simulink model "Takeoff_Sim"  (R2024a)
settings: Solver=ode4  StartTime=0.0  StopTime=15  FixedStep=0.01  RelTol=1e-3
values from neighbouring files (symbols this model uses):
  alpha_L0 = deg2rad(-2)    [Takeoff_Script.m]
  carrier_vel = 25 * 0.5144444444    (= 12.86111111)    [Takeoff_Script.m]
  CD_0 = 0.025    [Takeoff_Script.m]
  CD_LG = 0.01    [Takeoff_Script.m]
  CL_alpha = 2 * pi * AR / (2 + sqrt(AR^2 + 4))    [Takeoff_Script.m]
  g_accel = 9.807    [Takeoff_Script.m]
  k_drag = 1.0 / (eswald * pi * AR)    [Takeoff_Script.m]
  mass = 14000    [Takeoff_Script.m]
  mu_friction_nobrake = 0.04    [Takeoff_Script.m]
  thrust = 10000 * g_accel    (= 98070)    [Takeoff_Script.m]
  wingarea = x(1)    [Takeoff_Script.m]
libraries: simulink_extras x5, aerolibasang x2, aerolibatmos2 x1
settings Model: Creator=mfarr  LastModifiedBy=mfarr
settings OptimizationCC: BlockReduction=off  DefaultParameterBehavior=Inlined  BufferReuse=off

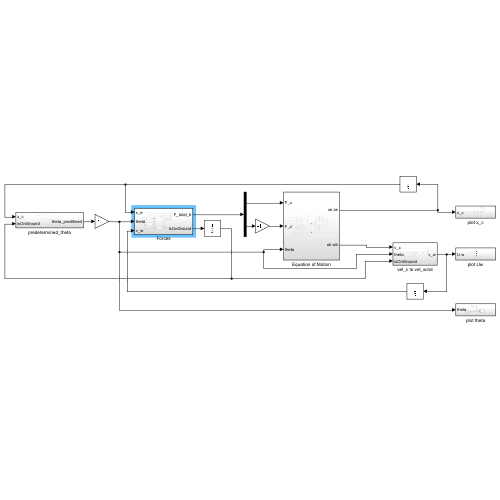
[thumbnail: Simulink's stored preview of the top-level diagram]
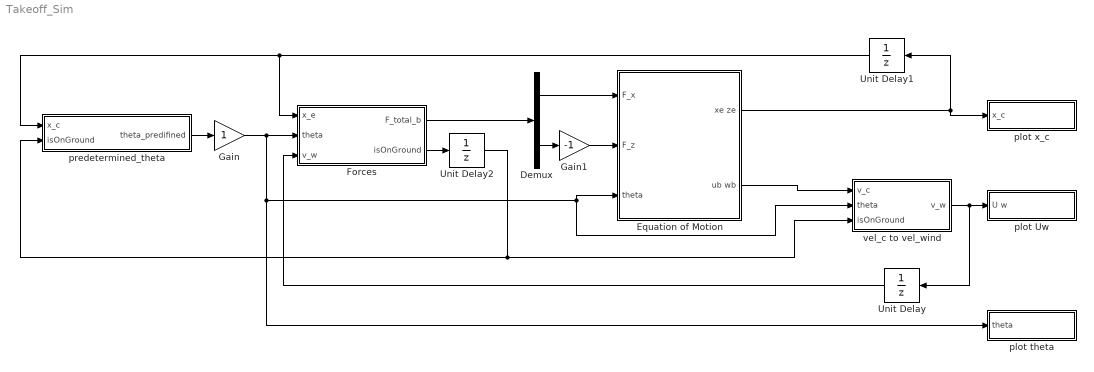
== system Takeoff_Sim ==
  Demux : Demux  Outputs=2
  Equation of Motion : Subsystem
  Forces : Subsystem
  Gain : Gain
  Gain1 : Gain  Gain=-1
  Unit Delay : UnitDelay  SampleTime=-1  HasFrameUpgradeWarning=on
  Unit Delay1 : UnitDelay  SampleTime=-1  HasFrameUpgradeWarning=on
  Unit Delay2 : UnitDelay  SampleTime=-1  HasFrameUpgradeWarning=on
  plot Uw : Subsystem
  plot theta : Subsystem
  plot x_c : Subsystem
  predetermined_theta : Subsystem
  vel_c to vel_wind : Subsystem
  wires:
  vel_c to vel_wind/1(v_w) -> Unit Delay/1, plot Uw/1(U w)
  Equation of Motion/2(ub wb) -> vel_c to vel_wind/1(v_c)
  Demux/1 -> Equation of Motion/1(F_x)
  Forces/1(F_total_b) -> Demux/1
  predetermined_theta/1(theta_predifined) -> Gain/1
  Unit Delay/1 -> Forces/3(v_w)
  Unit Delay1/1 -> predetermined_theta/1(x_c), Forces/1(x_e)
  Forces/2(isOnGround) -> Unit Delay2/1
  Unit Delay2/1 -> predetermined_theta/2(isOnGround), vel_c to vel_wind/3(isOnGround)
  Gain/1 -> Forces/2(theta), vel_c to vel_wind/2(theta), Equation of Motion/3(theta), plot theta/1(theta)
  Demux/2 -> Gain1/1
  Gain1/1 -> Equation of Motion/2(F_z)
  Equation of Motion/1(xe ze) -> plot x_c/1(x_c), Unit Delay1/1

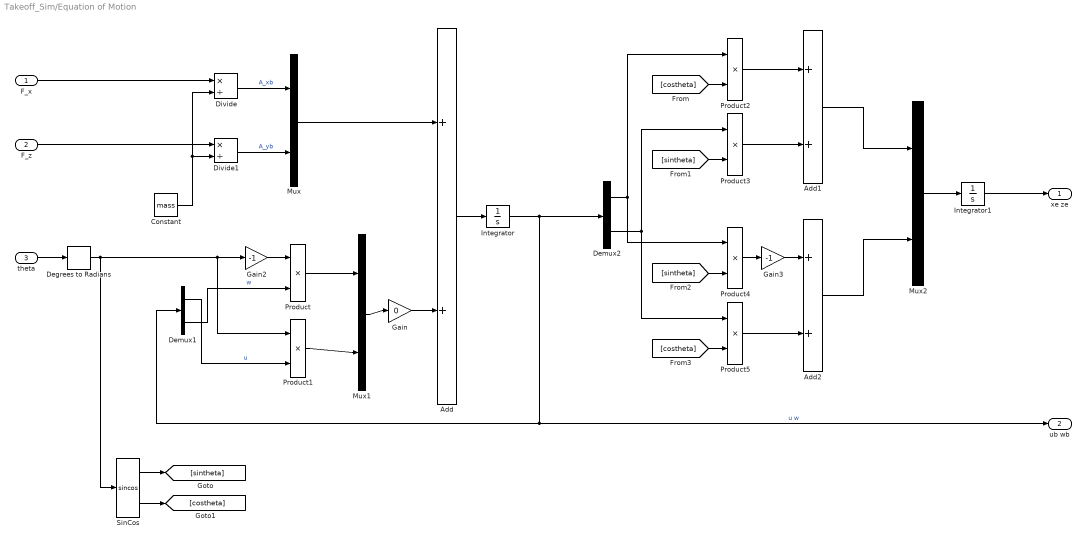
== system Takeoff_Sim/Equation of Motion ==
  F_x : Inport
  F_z : Inport  Port=2
  theta : Inport  Port=3
  Add : Sum
  Add1 : Sum
  Add2 : Sum
  Constant : Constant  Value=mass
  Degrees to Radians : simulink_extras/Transformations/Degrees to Radians
  Demux1 : Demux  Outputs=2
  Demux2 : Demux  Outputs=2
  Divide : Product  Inputs=*/  RndMeth=Zero  SaturateOnIntegerOverflow=on
  Divide1 : Product  Inputs=*/  RndMeth=Zero  SaturateOnIntegerOverflow=on
  Gain : Gain  Gain=0
  Gain2 : Gain  Gain=-1
  Gain3 : Gain  Gain=-1
  Integrator : Integrator
  Integrator1 : Integrator
  Mux : Mux  Inputs=2
  Mux1 : Mux  Inputs=2
  Mux2 : Mux  Inputs=2
  Product{,1..5} (6 alike) : Product
  SinCos : Trigonometry  Operator=sincos
  xe ze : Outport
  ub wb : Outport  Port=2
  wires:
  Demux1/2 -> Product/2  "w"
  Add1/1 -> Mux2/1
  SinCos/2 -> [costheta]
  Degrees to Radians/1 -> Product1/1, Gain2/1, SinCos/1
  Gain2/1 -> Product/1
  Divide1/1 -> Mux/2  "A_yb"
  Add/1 -> Integrator/1
  Mux/1 -> Add/1
  Demux1/1 -> Product1/2  "u"
  theta/1 -> Degrees to Radians/1
  Integrator/1 -> Demux2/1, ub wb/1, Demux1/1  "u w"
  Product5/1 -> Add2/2
  [costheta] -> Product5/2
  [costheta] -> Product2/2
  Product4/1 -> Gain3/1
  Mux1/1 -> Gain/1
  Constant/1 -> Divide1/2, Divide/2
  Demux2/2 -> Product3/1, Product5/1
  Divide/1 -> Mux/1  "A_xb"
  Mux2/1 -> Integrator1/1
  F_z/1 -> Divide1/1
  SinCos/1 -> [sintheta]
  [sintheta] -> Product3/2
  Demux2/1 -> Product4/1, Product2/1
  Gain3/1 -> Add2/1
  [sintheta] -> Product4/2
  Product3/1 -> Add1/2
  Integrator1/1 -> xe ze/1
  Product1/1 -> Mux1/2
  Product/1 -> Mux1/1
  Product2/1 -> Add1/1
  Add2/1 -> Mux2/2
  F_x/1 -> Divide/1
  Gain/1 -> Add/2

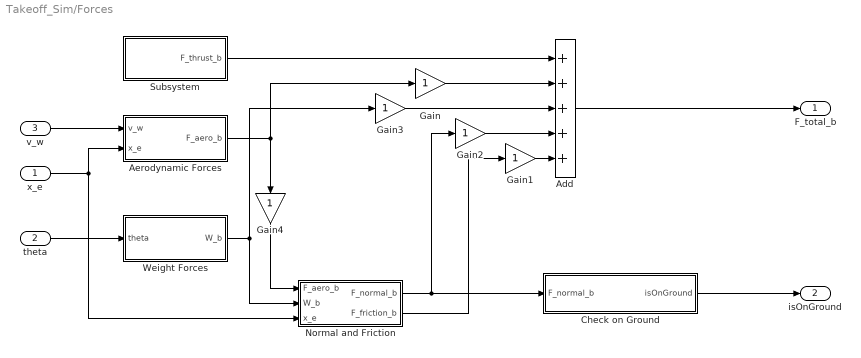
== system Takeoff_Sim/Forces ==
  x_e : Inport
  theta : Inport  Port=2
  v_w : Inport  Port=3
  Add : Sum  Inputs=+++++
  Aerodynamic Forces : Subsystem
  Check on Ground : Subsystem
  Gain{,1..4} (5 alike) : Gain
  Normal and Friction : Subsystem
  Subsystem : Subsystem
  Weight Forces : Subsystem
  F_total_b : Outport
  isOnGround : Outport  Port=2
  wires:
  Aerodynamic Forces/1(F_aero_b) -> Gain/1, Gain4/1
  Weight Forces/1(W_b) -> Gain3/1, Normal and Friction/2(W_b)
  theta/1 -> Weight Forces/1(theta)
  v_w/1 -> Aerodynamic Forces/1(v_w)
  x_e/1 -> Normal and Friction/3(x_e), Aerodynamic Forces/2(x_e)
  Add/1 -> F_total_b/1
  Subsystem/1(F_thrust_b) -> Add/1
  Normal and Friction/1(F_normal_b) -> Check on Ground/1(F_normal_b), Gain2/1
  Normal and Friction/2(F_friction_b) -> Gain1/1
  Gain/1 -> Add/2
  Gain1/1 -> Add/5
  Gain2/1 -> Add/4
  Gain3/1 -> Add/3
  Check on Ground/1(isOnGround) -> isOnGround/1
  Gain4/1 -> Normal and Friction/1(F_aero_b)

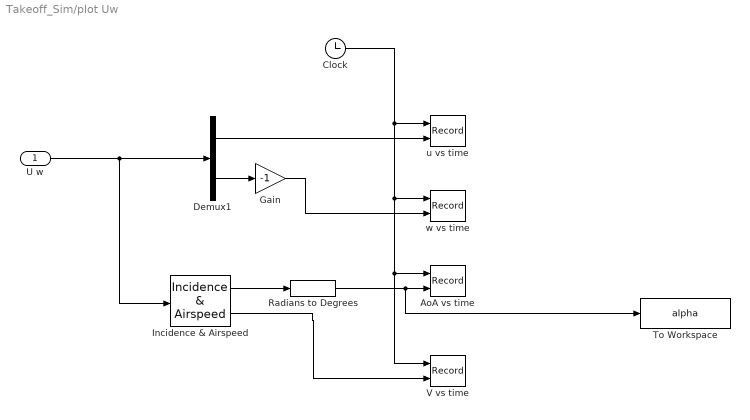
== system Takeoff_Sim/plot Uw ==
  U w : Inport
  AoA vs time : Record  FileSettingsInternal="{\"entries\":[{\"content\":{\"excelSettings\":{\"content\":{},\"type\":\"Streamout.ExcelSettings\"}},\"type\":\"Streamout.FileSettingStorage\",\"uuid\":\"\"}],\"packageUris\":[\"http:\\/\\/schema.mathworks.com\\/mf0\\/streamout_blocks\\/R2020a\"],\"version\":\"1.0\"}"  Layout=[1 1]  SignalsInternal="{\"entries\":[{\"content\":{\"signals\":[{\"content\":{\"blockPath\":[],\"dimensions\":[1],\"domain\":\"\",\"lineColor\":\"#a2142f\",\"plots\":[ 1 ],\"port\":1,\"sid\":[\"\"],\"signalID\":1,\"signalName\":\"Clock\"},\"type\":\"RecordBlkView.Signal\",\"uuid\":\"\"},{\"content\":{\"blockPath\":[],\"dimensions\":[1],\"domain\":\"\",\"lineColor\":\"#139fff\",\"plots\":[ 1 ],\"port\":2,\"sid\":[\"\"],\"signalID\":2,\"signalName\":\"Radians\\nto Degrees\"},\"type\":\"RecordBlkView.Signal\",\"uuid\":\"\"}]},\"type\":\"RecordBlkView.InputSignals\",\"uuid\":\"\"}],\"packageUris\":[\"http:\\/\\/schema.mathworks.com\\/mf0\\/streamout_blocks\\/R2020a\"],\"version\":\"1.0\"}"  VisualizationBindings="{\"xyplotplugin\":{\"info\":[{\"series\":[{\"bindingParametersList\":[{\"parameter\":\"X-Axis\",\"signalID\":1,\"signalName\":\"Clock\"},{\"parameter\":\"Y-Axis\",\"signalID\":2,\"signalName\":\"Radians\\nto Degrees\"}],\"seriesID\":0}],\"subplotID\":1}]}}"  CompatibilityTag=XY
  Clock : Clock
  Demux1 : Demux  Outputs=2
  Gain : Gain  Gain=-1
  Incidence & Airspeed : aerolibasang/Incidence  & Airspeed
  Radians to Degrees : simulink_extras/Transformations/Radians to Degrees
  To Workspace : ToWorkspace  VariableName=alpha  SampleTime=-1
      settings: Save2DSignal=2-D array (concatenate along first dimension)
  V vs time : Record  FileSettingsInternal="{\"entries\":[{\"content\":{\"excelSettings\":{\"content\":{},\"type\":\"Streamout.ExcelSettings\"}},\"type\":\"Streamout.FileSettingStorage\",\"uuid\":\"\"}],\"packageUris\":[\"http:\\/\\/schema.mathworks.com\\/mf0\\/streamout_blocks\\/R2020a\"],\"version\":\"1.0\"}"  Layout=[1 1]  SignalsInternal="{\"entries\":[{\"content\":{\"signals\":[{\"content\":{\"blockPath\":[],\"dimensions\":[1],\"domain\":\"\",\"lineColor\":\"#a2142f\",\"plots\":[ 1 ],\"port\":1,\"sid\":[\"\"],\"signalID\":1,\"signalName\":\"Clock\"},\"type\":\"RecordBlkView.Signal\",\"uuid\":\"\"},{\"content\":{\"blockPath\":[],\"dimensions\":[1],\"domain\":\"\",\"lineColor\":\"#139fff\",\"plots\":[ 1 ],\"port\":2,\"sid\":[\"\"],\"signalID\":2,\"signalName\":\"Incidence \\n& Airspeed:2\"},\"type\":\"RecordBlkView.Signal\",\"uuid\":\"\"}]},\"type\":\"RecordBlkView.InputSignals\",\"uuid\":\"\"}],\"packageUris\":[\"http:\\/\\/schema.mathworks.com\\/mf0\\/streamout_blocks\\/R2020a\"],\"version\":\"1.0\"}"  VisualizationBindings="{\"xyplotplugin\":{\"info\":[{\"series\":[{\"bindingParametersList\":[{\"parameter\":\"X-Axis\",\"signalID\":1,\"signalName\":\"Clock\"},{\"parameter\":\"Y-Axis\",\"signalID\":2,\"signalName\":\"Incidence \\n& Airspeed:2\"}],\"seriesID\":0}],\"subplotID\":1}]}}"  CompatibilityTag=XY
  u vs time : Record  FileSettingsInternal="{\"entries\":[{\"content\":{\"excelSettings\":{\"content\":{},\"type\":\"Streamout.ExcelSettings\"}},\"type\":\"Streamout.FileSettingStorage\",\"uuid\":\"\"}],\"packageUris\":[\"http:\\/\\/schema.mathworks.com\\/mf0\\/streamout_blocks\\/R2020a\"],\"version\":\"1.0\"}"  Layout=[1 1]  SignalsInternal="{\"entries\":[{\"content\":{\"signals\":[{\"content\":{\"blockPath\":[],\"dimensions\":[1],\"domain\":\"\",\"lineColor\":\"#a2142f\",\"plots\":[ 1 ],\"port\":1,\"sid\":[\"\"],\"signalID\":1,\"signalName\":\"Clock\"},\"type\":\"RecordBlkView.Signal\",\"uuid\":\"\"},{\"content\":{\"blockPath\":[],\"dimensions\":[1],\"domain\":\"\",\"lineColor\":\"#139fff\",\"plots\":[ 1 ],\"port\":2,\"sid\":[\"\"],\"signalID\":2,\"signalName\":\"Demux1:1\"},\"type\":\"RecordBlkView.Signal\",\"uuid\":\"\"}]},\"type\":\"RecordBlkView.InputSignals\",\"uuid\":\"\"}],\"packageUris\":[\"http:\\/\\/schema.mathworks.com\\/mf0\\/streamout_blocks\\/R2020a\"],\"version\":\"1.0\"}"  VisualizationBindings="{\"xyplotplugin\":{\"info\":[{\"series\":[{\"bindingParametersList\":[{\"parameter\":\"X-Axis\",\"signalID\":1,\"signalName\":\"Clock\"},{\"parameter\":\"Y-Axis\",\"signalID\":2,\"signalName\":\"Demux1:1\"}],\"seriesID\":0}],\"subplotID\":1}]}}"  CompatibilityTag=XY
  w vs time : Record  FileSettingsInternal="{\"entries\":[{\"content\":{\"excelSettings\":{\"content\":{},\"type\":\"Streamout.ExcelSettings\"}},\"type\":\"Streamout.FileSettingStorage\",\"uuid\":\"\"}],\"packageUris\":[\"http:\\/\\/schema.mathworks.com\\/mf0\\/streamout_blocks\\/R2020a\"],\"version\":\"1.0\"}"  Layout=[1 1]  SignalsInternal="{\"entries\":[{\"content\":{\"signals\":[{\"content\":{\"blockPath\":[],\"dimensions\":[1],\"domain\":\"\",\"lineColor\":\"#a2142f\",\"plots\":[ 1 ],\"port\":1,\"sid\":[\"\"],\"signalID\":1,\"signalName\":\"Clock\"},\"type\":\"RecordBlkView.Signal\",\"uuid\":\"\"},{\"content\":{\"blockPath\":[],\"dimensions\":[1],\"domain\":\"\",\"lineColor\":\"#139fff\",\"plots\":[ 1 ],\"port\":2,\"sid\":[\"\"],\"signalID\":2,\"signalName\":\"Gain\"},\"type\":\"RecordBlkView.Signal\",\"uuid\":\"\"}]},\"type\":\"RecordBlkView.InputSignals\",\"uuid\":\"\"}],\"packageUris\":[\"http:\\/\\/schema.mathworks.com\\/mf0\\/streamout_blocks\\/R2020a\"],\"version\":\"1.0\"}"  VisualizationBindings="{\"xyplotplugin\":{\"info\":[{\"series\":[{\"bindingParametersList\":[{\"parameter\":\"X-Axis\",\"signalID\":1,\"signalName\":\"Clock\"},{\"parameter\":\"Y-Axis\",\"signalID\":2,\"signalName\":\"Gain\"}],\"seriesID\":0}],\"subplotID\":1}]}}"  CompatibilityTag=XY
  wires:
  U w/1 -> Incidence & Airspeed/1, Demux1/1
  Clock/1 -> u vs time/1, w vs time/1, V vs time/1, AoA vs time/1
  Demux1/2 -> Gain/1
  Gain/1 -> w vs time/2
  Demux1/1 -> u vs time/2
  Incidence & Airspeed/1 -> Radians to Degrees/1
  Radians to Degrees/1 -> To Workspace/1, AoA vs time/2
  Incidence & Airspeed/2 -> V vs time/2

== system Takeoff_Sim/plot theta ==
  theta : Inport
  Clock : Clock
  theta vs time : Record  FileSettingsInternal="{\"entries\":[{\"content\":{\"excelSettings\":{\"content\":{},\"type\":\"Streamout.ExcelSettings\"}},\"type\":\"Streamout.FileSettingStorage\",\"uuid\":\"\"}],\"packageUris\":[\"http:\\/\\/schema.mathworks.com\\/mf0\\/streamout_blocks\\/R2020a\"],\"version\":\"1.0\"}"  Layout=[1 1]  SignalsInternal="{\"entries\":[{\"content\":{\"signals\":[{\"content\":{\"blockPath\":[],\"dimensions\":[1],\"domain\":\"\",\"lineColor\":\"#a2142f\",\"plots\":[ 1 ],\"port\":1,\"sid\":[\"\"],\"signalID\":1,\"signalName\":\"Clock\"},\"type\":\"RecordBlkView.Signal\",\"uuid\":\"\"},{\"content\":{\"blockPath\":[],\"dimensions\":[1],\"domain\":\"\",\"lineColor\":\"#139fff\",\"plots\":[ 1 ],\"port\":2,\"sid\":[\"\"],\"signalID\":2,\"signalName\":\"theta\"},\"type\":\"RecordBlkView.Signal\",\"uuid\":\"\"}]},\"type\":\"RecordBlkView.InputSignals\",\"uuid\":\"\"}],\"packageUris\":[\"http:\\/\\/schema.mathworks.com\\/mf0\\/streamout_blocks\\/R2020a\"],\"version\":\"1.0\"}"  VisualizationBindings="{\"xyplotplugin\":{\"info\":[{\"series\":[{\"bindingParametersList\":[{\"parameter\":\"X-Axis\",\"signalID\":1,\"signalName\":\"Clock\"},{\"parameter\":\"Y-Axis\",\"signalID\":2,\"signalName\":\"theta\"}],\"seriesID\":0}],\"subplotID\":1}]}}"  CompatibilityTag=XY
  wires:
  theta/1 -> theta vs time/2
  Clock/1 -> theta vs time/1

== system Takeoff_Sim/plot x_c ==
  x_c : Inport
  Demux1 : Demux  Outputs=2
  Gain : Gain  Gain=-1
  To Workspace : ToWorkspace  VariableName=x_c  SampleTime=-1
      settings: Save2DSignal=2-D array (concatenate along first dimension)
  To Workspace1 : ToWorkspace  VariableName=y_c  SampleTime=-1
      settings: Save2DSignal=2-D array (concatenate along first dimension)
  XY Graph : Record  FileSettingsInternal="{\"entries\":[{\"content\":{\"excelSettings\":{\"content\":{},\"type\":\"Streamout.ExcelSettings\"}},\"type\":\"Streamout.FileSettingStorage\",\"uuid\":\"\"}],\"packageUris\":[\"http:\\/\\/schema.mathworks.com\\/mf0\\/streamout_blocks\\/R2020a\"],\"version\":\"1.0\"}"  Layout=[1 1]  SignalsInternal="{\"entries\":[{\"content\":{\"signals\":[{\"content\":{\"blockPath\":[],\"dimensions\":[1],\"domain\":\"\",\"lineColor\":\"#64d413\",\"lineWidth\":2,\"plots\":[ 1 ],\"port\":1,\"sid\":[\"\"],\"signalID\":1,\"signalName\":\"Demux1:1\"},\"type\":\"RecordBlkView.Signal\",\"uuid\":\"\"},{\"content\":{\"blockPath\":[],\"dimensions\":[1],\"domain\":\"\",\"lineColor\":\"#ff13a6\",\"lineWidth\":2,\"plots\":[ 1 ],\"port\":2,\"sid\":[\"\"],\"signalID\":2,\"signalName\":\"Gain\"},\"type\":\"RecordBlkView.Signal\",\"uuid\":\"\"}]},\"type\":\"RecordBlkView.InputSignals\",\"uuid\":\"\"}],\"packageUris\":[\"http:\\/\\/schema.mathworks.com\\/mf0\\/streamout_blocks\\/R2020a\"],\"version\":\"1.0\"}"  VisualizationBindings="{\"xyplotplugin\":{\"info\":[{\"series\":[{\"bindingParametersList\":[{\"parameter\":\"X-Axis\",\"signalID\":1,\"signalName\":\"Demux1:1\"},{\"parameter\":\"Y-Axis\",\"signalID\":2,\"signalName\":\"Gain\"}],\"seriesID\":0}],\"subplotID\":1}]}}"  CompatibilityTag=XY
  wires:
  x_c/1 -> Demux1/1
  Demux1/2 -> Gain/1
  Demux1/1 -> To Workspace/1, XY Graph/1
  Gain/1 -> XY Graph/2, To Workspace1/1

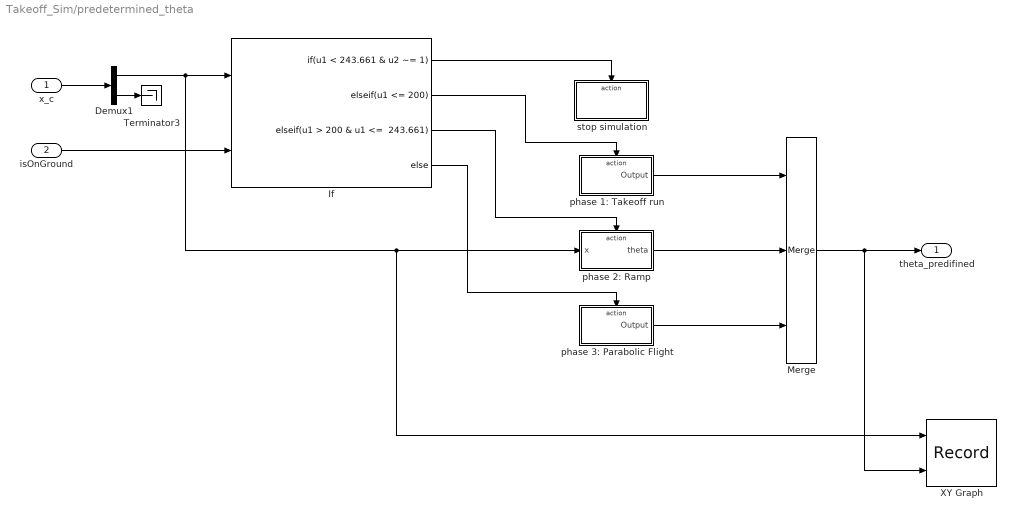
== system Takeoff_Sim/predetermined_theta ==
  x_c : Inport
  isOnGround : Inport  Port=2
  Demux1 : Demux  Outputs=2
  If : If  NumInputs=2  IfExpression=u1 < 243.661 & u2 ~= 1  ElseIfExpressions="u1 <= 200, u1 > 200 & u1 <=  243.661"
  Merge : Merge  Inputs=3
  Terminator3 : Terminator
  XY Graph : Record  FileSettingsInternal="{\"entries\":[{\"content\":{\"excelSettings\":{\"content\":{},\"type\":\"Streamout.ExcelSettings\"}},\"type\":\"Streamout.FileSettingStorage\",\"uuid\":\"\"}],\"packageUris\":[\"http:\\/\\/schema.mathworks.com\\/mf0\\/streamout_blocks\\/R2020a\"],\"version\":\"1.0\"}"  Layout=[1 1]  SignalsInternal="{\"entries\":[{\"content\":{\"signals\":[{\"content\":{\"blockPath\":[],\"dimensions\":[1],\"domain\":\"\",\"lineColor\":\"#a2142f\",\"plots\":[ 1 ],\"port\":1,\"sid\":[\"\"],\"signalID\":1,\"signalName\":\"Demux1:1\"},\"type\":\"RecordBlkView.Signal\",\"uuid\":\"\"},{\"content\":{\"blockPath\":[],\"dimensions\":[1],\"domain\":\"\",\"lineColor\":\"#139fff\",\"plots\":[ 1 ],\"port\":2,\"sid\":[\"\"],\"signalID\":2,\"signalName\":\"Merge\"},\"type\":\"RecordBlkView.Signal\",\"uuid\":\"\"}]},\"type\":\"RecordBlkView.InputSignals\",\"uuid\":\"\"}],\"packageUris\":[\"http:\\/\\/schema.mathworks.com\\/mf0\\/streamout_blocks\\/R2020a\"],\"version\":\"1.0\"}"  VisualizationBindings="{\"xyplotplugin\":{\"info\":[{\"series\":[{\"bindingParametersList\":[{\"parameter\":\"X-Axis\",\"signalID\":1,\"signalName\":\"Demux1:1\"},{\"parameter\":\"Y-Axis\",\"signalID\":2,\"signalName\":\"Merge\"}],\"seriesID\":0}],\"subplotID\":1}]}}"  CompatibilityTag=XY
  phase 1: Takeoff run : Subsystem  TreatAsAtomicUnit=on
  phase 2: Ramp : Subsystem  TreatAsAtomicUnit=on
  phase 3: Parabolic Flight : Subsystem  TreatAsAtomicUnit=on
  stop simulation : Subsystem  TreatAsAtomicUnit=on
  theta_predifined : Outport
  wires:
  isOnGround/1 -> If/2
  phase 2: Ramp/1(theta) -> Merge/2
  If/2 -> phase 1: Takeoff run/Action
  x_c/1 -> Demux1/1
  Demux1/1 -> XY Graph/1, phase 2: Ramp/1(x), If/1
  Demux1/2 -> Terminator3/1
  If/4 -> phase 3: Parabolic Flight/Action
  If/3 -> phase 2: Ramp/Action
  If/1 -> stop simulation/Action
  Merge/1 -> XY Graph/2, theta_predifined/1
  phase 1: Takeoff run/1(Output) -> Merge/1
  phase 3: Parabolic Flight/1(Output) -> Merge/3

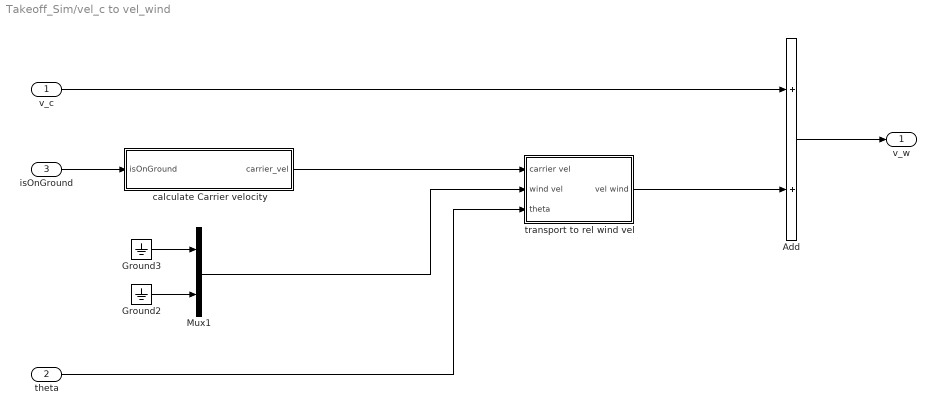
== system Takeoff_Sim/vel_c to vel_wind ==
  v_c : Inport
  theta : Inport  Port=2
  isOnGround : Inport  Port=3
  Add : Sum
  Ground2 : Ground
  Ground3 : Ground
  Mux1 : Mux  Inputs=2
  calculate Carrier velocity : Subsystem
  transport to rel wind vel : Subsystem
  v_w : Outport  PortDimensions=2
  wires:
  Ground3/1 -> Mux1/1
  Ground2/1 -> Mux1/2
  isOnGround/1 -> calculate Carrier velocity/1(isOnGround)
  calculate Carrier velocity/1(carrier_vel) -> transport to rel wind vel/1(carrier vel)
  Mux1/1 -> transport to rel wind vel/2(wind vel)
  theta/1 -> transport to rel wind vel/3(theta)
  v_c/1 -> Add/1
  transport to rel wind vel/1(vel wind) -> Add/2
  Add/1 -> v_w/1

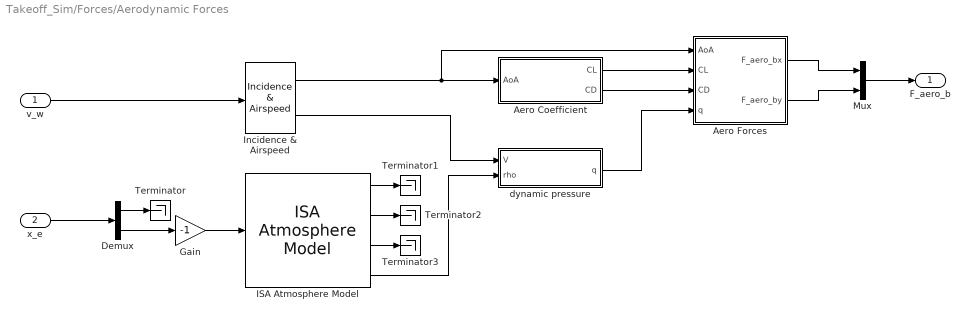
== system Takeoff_Sim/Forces/Aerodynamic Forces ==
  v_w : Inport
  x_e : Inport  Port=2
  Aero Coefficient : Subsystem
  Aero Forces : Subsystem
  Demux : Demux  Outputs=2
  Gain : Gain  Gain=-1
  ISA Atmosphere Model : aerolibatmos2/ISA Atmosphere Model  useExtended=off  action=Warning  custom=off  viscosityOut=off  g=9.80665  gamma=1.4  R=287.0531  L=0.0065  h_trop=11000  h_strat=20000  rho0=1.225  P0=101325  T0=288.15  h0=0  S=110.4  Tref=273.15  muref=1.716e-5
  Incidence & Airspeed : aerolibasang/Incidence  & Airspeed
  Mux : Mux  Inputs=2
  Terminator{,1..3} (4 alike) : Terminator
  dynamic pressure : Subsystem
  F_aero_b : Outport
  wires:
  Mux/1 -> F_aero_b/1
  x_e/1 -> Demux/1
  Demux/1 -> Terminator/1
  Demux/2 -> Gain/1
  Gain/1 -> ISA Atmosphere Model/1
  v_w/1 -> Incidence & Airspeed/1
  ISA Atmosphere Model/1 -> Terminator1/1
  ISA Atmosphere Model/2 -> Terminator2/1
  ISA Atmosphere Model/3 -> Terminator3/1
  Incidence & Airspeed/1 -> Aero Forces/1(AoA), Aero Coefficient/1(AoA)
  Aero Coefficient/1(CL) -> Aero Forces/2(CL)
  Aero Coefficient/2(CD) -> Aero Forces/3(CD)
  Aero Forces/1(F_aero_bx) -> Mux/1
  Aero Forces/2(F_aero_by) -> Mux/2
  Incidence & Airspeed/2 -> dynamic pressure/1(V)
  ISA Atmosphere Model/4 -> dynamic pressure/2(rho)
  dynamic pressure/1(q) -> Aero Forces/4(q)

== system Takeoff_Sim/Forces/Check on Ground ==
  F_normal_b : Inport
  Aircraft on Air : Subsystem  TreatAsAtomicUnit=on
  Aircraft on Ground : Subsystem  TreatAsAtomicUnit=on
  Clock : Clock
  If : If
  Merge : Merge
  XY Graph : Record  FileSettingsInternal="{\"entries\":[{\"content\":{\"excelSettings\":{\"content\":{},\"type\":\"Streamout.ExcelSettings\"}},\"type\":\"Streamout.FileSettingStorage\",\"uuid\":\"\"}],\"packageUris\":[\"http:\\/\\/schema.mathworks.com\\/mf0\\/streamout_blocks\\/R2020a\"],\"version\":\"1.0\"}"  Layout=[1 1]  SignalsInternal="{\"entries\":[{\"content\":{\"signals\":[{\"content\":{\"blockPath\":[],\"dimensions\":[1],\"domain\":\"\",\"lineColor\":\"#a2142f\",\"plots\":[ 1 ],\"port\":1,\"sid\":[\"\"],\"signalID\":1,\"signalName\":\"Clock\"},\"type\":\"RecordBlkView.Signal\",\"uuid\":\"\"},{\"content\":{\"blockPath\":[],\"dimensions\":[1],\"domain\":\"\",\"lineColor\":\"#139fff\",\"plots\":[ 1 ],\"port\":2,\"sid\":[\"\"],\"signalID\":2,\"signalName\":\"Merge\"},\"type\":\"RecordBlkView.Signal\",\"uuid\":\"\"}]},\"type\":\"RecordBlkView.InputSignals\",\"uuid\":\"\"}],\"packageUris\":[\"http:\\/\\/schema.mathworks.com\\/mf0\\/streamout_blocks\\/R2020a\"],\"version\":\"1.0\"}"  VisualizationBindings="{\"xyplotplugin\":{\"info\":[{\"series\":[{\"bindingParametersList\":[{\"parameter\":\"X-Axis\",\"signalID\":1,\"signalName\":\"Clock\"},{\"parameter\":\"Y-Axis\",\"signalID\":2,\"signalName\":\"Merge\"}],\"seriesID\":0}],\"subplotID\":1}]}}"  CompatibilityTag=XY
  isOnGround : Outport
  wires:
  If/1 -> Aircraft on Ground/Action
  Aircraft on Air/1(isOnGround) -> Merge/2
  If/2 -> Aircraft on Air/Action
  Aircraft on Ground/1(isOnGround) -> Merge/1
  F_normal_b/1 -> If/1
  Clock/1 -> XY Graph/1
  Merge/1 -> XY Graph/2, isOnGround/1

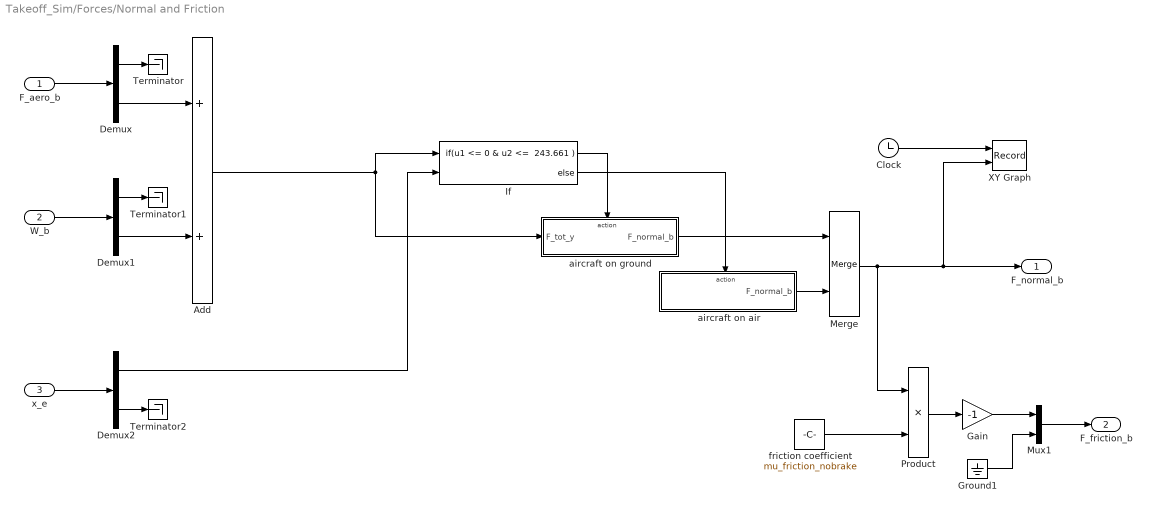
== system Takeoff_Sim/Forces/Normal and Friction ==
  F_aero_b : Inport
  W_b : Inport  Port=2
  x_e : Inport  Port=3
  Add : Sum
  Clock : Clock
  Demux : Demux  Outputs=2
  Demux1 : Demux  Outputs=2
  Demux2 : Demux  Outputs=2
  Gain : Gain  Gain=-1
  Ground1 : Ground
  If : If  NumInputs=2  IfExpression="u1 <= 0 & u2 <=  243.661"
  Merge : Merge
  Mux1 : Mux  Inputs=2
  Product : Product
  Terminator : Terminator
  Terminator1 : Terminator
  Terminator2 : Terminator
  XY Graph : Record  FileSettingsInternal="{\"entries\":[{\"content\":{\"excelSettings\":{\"content\":{},\"type\":\"Streamout.ExcelSettings\"}},\"type\":\"Streamout.FileSettingStorage\",\"uuid\":\"\"}],\"packageUris\":[\"http:\\/\\/schema.mathworks.com\\/mf0\\/streamout_blocks\\/R2020a\"],\"version\":\"1.0\"}"  Layout=[1 1]  SignalsInternal="{\"entries\":[{\"content\":{\"signals\":[{\"content\":{\"blockPath\":[],\"dimensions\":[1],\"domain\":\"\",\"lineColor\":\"#a2142f\",\"plots\":[ 1 ],\"port\":1,\"sid\":[\"\"],\"signalID\":1,\"signalName\":\"Clock\"},\"type\":\"RecordBlkView.Signal\",\"uuid\":\"\"},{\"content\":{\"blockPath\":[],\"dimensions\":[1],\"domain\":\"\",\"lineColor\":\"#139fff\",\"plots\":[ 1 ],\"port\":2,\"sid\":[\"\"],\"signalID\":2,\"signalName\":\"Merge\"},\"type\":\"RecordBlkView.Signal\",\"uuid\":\"\"}]},\"type\":\"RecordBlkView.InputSignals\",\"uuid\":\"\"}],\"packageUris\":[\"http:\\/\\/schema.mathworks.com\\/mf0\\/streamout_blocks\\/R2020a\"],\"version\":\"1.0\"}"  VisualizationBindings="{\"xyplotplugin\":{\"info\":[{\"series\":[{\"bindingParametersList\":[{\"parameter\":\"X-Axis\",\"signalID\":1,\"signalName\":\"Clock\"},{\"parameter\":\"Y-Axis\",\"signalID\":2,\"signalName\":\"Merge\"}],\"seriesID\":0}],\"subplotID\":1}]}}"  CompatibilityTag=XY
  aircraft on air : Subsystem  TreatAsAtomicUnit=on
  aircraft on ground : Subsystem  TreatAsAtomicUnit=on
  friction coefficient : Constant  Value=mu_friction_nobrake
  F_normal_b : Outport
  F_friction_b : Outport  Port=2
  wires:
  Merge/1 -> Product/1, XY Graph/2, F_normal_b/1
  Mux1/1 -> F_friction_b/1
  F_aero_b/1 -> Demux/1
  Demux/1 -> Terminator/1
  W_b/1 -> Demux1/1
  Demux1/1 -> Terminator1/1
  Demux/2 -> Add/1
  Demux1/2 -> Add/2
  Add/1 -> If/1, aircraft on ground/1(F_tot_y)
  If/2 -> aircraft on air/Action
  friction coefficient/1 -> Product/2
  Product/1 -> Gain/1
  Gain/1 -> Mux1/1
  Ground1/1 -> Mux1/2
  aircraft on air/1(F_normal_b) -> Merge/2
  aircraft on ground/1(F_normal_b) -> Merge/1
  Clock/1 -> XY Graph/1
  x_e/1 -> Demux2/1
  Demux2/2 -> Terminator2/1
  Demux2/1 -> If/2
  If/1 -> aircraft on ground/Action

== system Takeoff_Sim/Forces/Subsystem ==
  Ground : Ground
  Mux : Mux  Inputs=2
  thrust : Constant  Value=thrust
  F_thrust_b : Outport
  wires:
  thrust/1 -> Mux/1
  Mux/1 -> F_thrust_b/1
  Ground/1 -> Mux/2

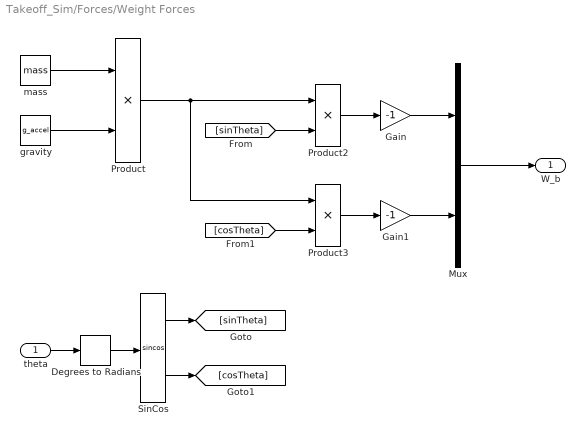
== system Takeoff_Sim/Forces/Weight Forces ==
  theta : Inport
  Degrees to Radians : simulink_extras/Transformations/Degrees to Radians
  Gain : Gain  Gain=-1
  Gain1 : Gain  Gain=-1
  Mux : Mux  Inputs=2
  Product : Product
  Product2 : Product
  Product3 : Product
  SinCos : Trigonometry  Operator=sincos
  gravity : Constant  Value=g_accel
  mass : Constant  Value=mass
  W_b : Outport
  wires:
  Mux/1 -> W_b/1
  [cosTheta] -> Product3/2
  [sinTheta] -> Product2/2
  Product/1 -> Product3/1, Product2/1
  mass/1 -> Product/1
  gravity/1 -> Product/2
  theta/1 -> Degrees to Radians/1
  Degrees to Radians/1 -> SinCos/1
  SinCos/1 -> [sinTheta]
  SinCos/2 -> [cosTheta]
  Product2/1 -> Gain/1
  Gain/1 -> Mux/1
  Product3/1 -> Gain1/1
  Gain1/1 -> Mux/2

== system Takeoff_Sim/predetermined_theta/phase 1: Takeoff run ==
  Action Port : ActionPort  ActionPortLabel=elseif(u1 <= 200)
  Constant : Constant  Value=0
  Output : Outport
  wires:
  Constant/1 -> Output/1

== system Takeoff_Sim/predetermined_theta/phase 2: Ramp ==
  x : Inport
  Action Port : ActionPort  ActionPortLabel="elseif( u1 > 200 & u1 <=  243.661 )"
  Constant : Constant  Value=210
  MATLAB Function : MATLAB Function  TreatAsAtomicUnit=on
  theta : Outport
  wires:
  x/1 -> MATLAB Function/1(x)
  Constant/1 -> MATLAB Function/2(R)
  MATLAB Function/1(theta) -> theta/1

== system Takeoff_Sim/predetermined_theta/phase 3: Parabolic Flight ==
  Action Port : ActionPort  ActionPortLabel=else
  Constant : Constant  Value=12
  Output : Outport
  wires:
  Constant/1 -> Output/1

== system Takeoff_Sim/predetermined_theta/stop simulation ==
  Action Port : ActionPort  ActionPortLabel=if(u1 < 243.661 & u2 ~= 1)
  Assertion : Assertion  AssertionFailFcn=Aircraft lift-off before the end of the runway
  Constant : Constant
  wires:
  Constant/1 -> Assertion/1

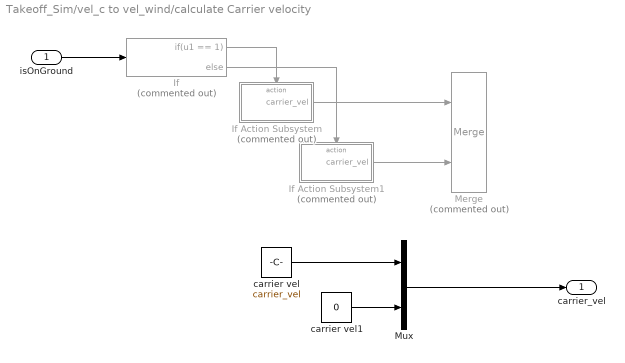
== system Takeoff_Sim/vel_c to vel_wind/calculate Carrier velocity ==
  isOnGround : Inport
  If : If  Commented=on  IfExpression=u1 == 1
  If Action Subsystem : Subsystem  Commented=on  TreatAsAtomicUnit=on
  If Action Subsystem1 : Subsystem  Commented=on  TreatAsAtomicUnit=on
  Merge : Merge  Commented=on
  Mux : Mux  Inputs=2
  carrier vel : Constant  Value=carrier_vel
  carrier vel1 : Constant  Value=0
  carrier_vel : Outport  PortDimensions=2
  wires:
  If/2 -> If Action Subsystem1/Action
  If Action Subsystem1/1(carrier_vel) -> Merge/2
  If/1 -> If Action Subsystem/Action
  If Action Subsystem/1(carrier_vel) -> Merge/1
  isOnGround/1 -> If/1
  carrier vel1/1 -> Mux/2
  carrier vel/1 -> Mux/1
  Mux/1 -> carrier_vel/1

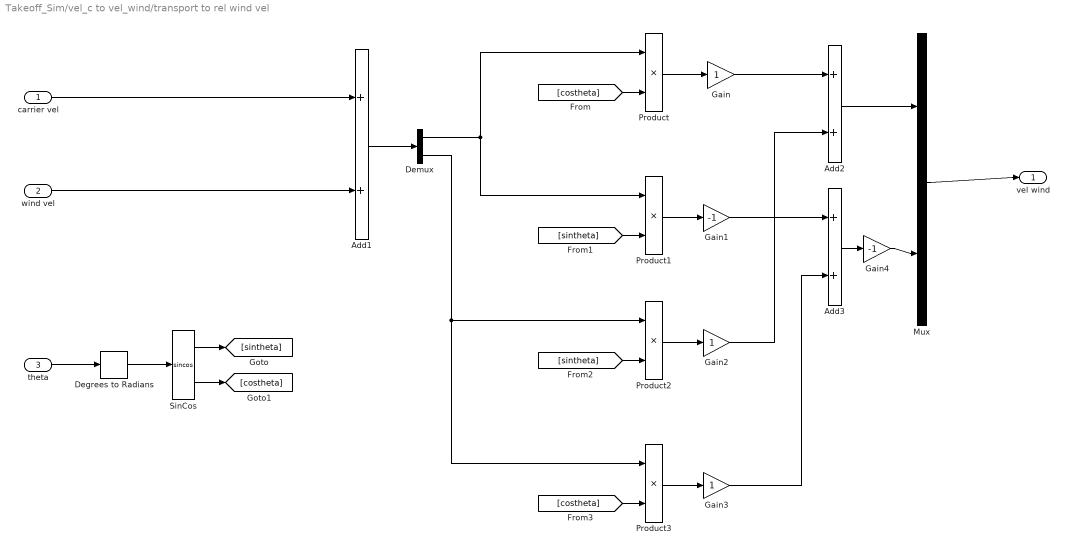
== system Takeoff_Sim/vel_c to vel_wind/transport to rel wind vel ==
  carrier vel : Inport
  wind vel : Inport  Port=2
  theta : Inport  Port=3
  Add1 : Sum
  Add2 : Sum
  Add3 : Sum
  Degrees to Radians : simulink_extras/Transformations/Degrees to Radians
  Demux : Demux  Outputs=2
  Gain : Gain
  Gain1 : Gain  Gain=-1
  Gain2 : Gain
  Gain3 : Gain
  Gain4 : Gain  Gain=-1
  Mux : Mux  Inputs=2
  Product{,1..3} (4 alike) : Product
  SinCos : Trigonometry  Operator=sincos
  vel wind : Outport
  wires:
  Gain1/1 -> Add3/1
  Gain2/1 -> Add2/2
  Demux/1 -> Product1/1, Product/1
  SinCos/1 -> [sintheta]
  wind vel/1 -> Add1/2
  [sintheta] -> Product2/2
  Demux/2 -> Product3/1, Product2/1
  Product3/1 -> Gain3/1
  Add3/1 -> Gain4/1
  Gain/1 -> Add2/1
  Gain3/1 -> Add3/2
  Degrees to Radians/1 -> SinCos/1
  Product/1 -> Gain/1
  [costheta] -> Product3/2
  Product2/1 -> Gain2/1
  Mux/1 -> vel wind/1
  Add1/1 -> Demux/1
  [sintheta] -> Product1/2
  [costheta] -> Product/2
  SinCos/2 -> [costheta]
  theta/1 -> Degrees to Radians/1
  carrier vel/1 -> Add1/1
  Add2/1 -> Mux/1
  Product1/1 -> Gain1/1
  Gain4/1 -> Mux/2

== system Takeoff_Sim/Forces/Aerodynamic Forces/Aero Coefficient ==
  AoA : Inport
  Calculate CD : Subsystem
  Calculate CL : Subsystem
  CL : Outport
  CD : Outport  Port=2
  wires:
  Calculate CD/1(CD) -> CD/1
  AoA/1 -> Calculate CL/1(AoA)
  Calculate CL/1(CL) -> CL/1, Calculate CD/1(CL)

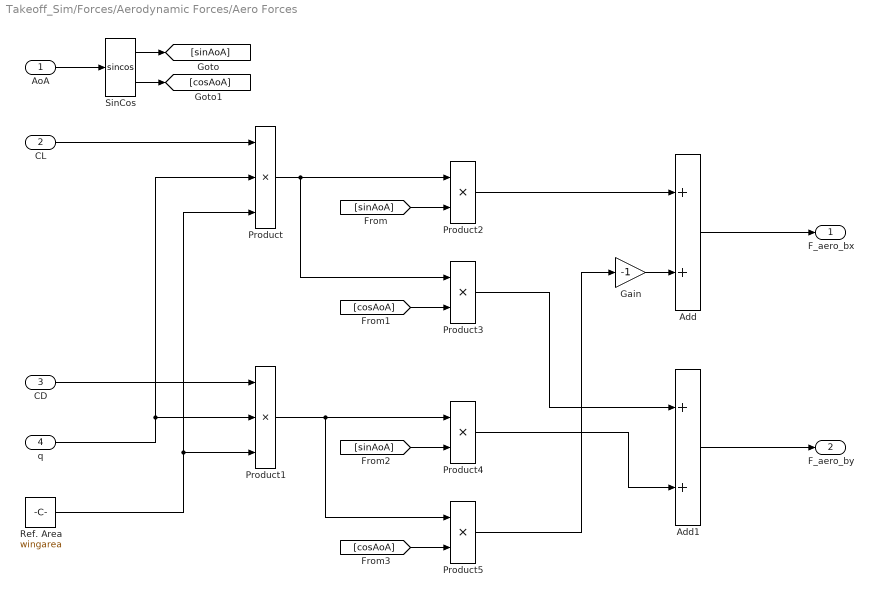
== system Takeoff_Sim/Forces/Aerodynamic Forces/Aero Forces ==
  AoA : Inport
  CL : Inport  Port=2
  CD : Inport  Port=3
  q : Inport  Port=4
  Add : Sum
  Add1 : Sum
  Gain : Gain  Gain=-1
  Product : Product  Inputs=3
  Product1 : Product  Inputs=3
  Product{2..5} (4 alike) : Product
  Ref. Area : Constant  Value=wingarea
  SinCos : Trigonometry  Operator=sincos
  F_aero_bx : Outport
  F_aero_by : Outport  Port=2
  wires:
  AoA/1 -> SinCos/1
  SinCos/1 -> [sinAoA]
  SinCos/2 -> [cosAoA]
  CL/1 -> Product/1
  q/1 -> Product1/2, Product/2
  Ref. Area/1 -> Product1/3, Product/3
  CD/1 -> Product1/1
  Product/1 -> Product3/1, Product2/1
  [sinAoA] -> Product2/2
  [cosAoA] -> Product3/2
  [cosAoA] -> Product5/2
  [sinAoA] -> Product4/2
  Product1/1 -> Product5/1, Product4/1
  Product2/1 -> Add/1
  Gain/1 -> Add/2
  Product5/1 -> Gain/1
  Add/1 -> F_aero_bx/1
  Product3/1 -> Add1/1
  Product4/1 -> Add1/2
  Add1/1 -> F_aero_by/1

== system Takeoff_Sim/Forces/Aerodynamic Forces/dynamic pressure ==
  V : Inport
  rho : Inport  Port=2
  Constant : Constant  Value=0.5
  Product : Product  Inputs=3
  Square : Math  Operator=square
  q : Outport
  wires:
  rho/1 -> Product/2
  Product/1 -> q/1
  Constant/1 -> Product/1
  Square/1 -> Product/3
  V/1 -> Square/1

== system Takeoff_Sim/Forces/Check on Ground/Aircraft on Air ==
  Action Port : ActionPort  ActionPortLabel=else
  Constant : Constant  Value=0
  isOnGround : Outport
  wires:
  Constant/1 -> isOnGround/1

== system Takeoff_Sim/Forces/Check on Ground/Aircraft on Ground ==
  Action Port : ActionPort  ActionPortLabel=if(u1 > 0)
  Constant : Constant
  isOnGround : Outport
  wires:
  Constant/1 -> isOnGround/1

== system Takeoff_Sim/Forces/Normal and Friction/aircraft on air ==
  Action Port : ActionPort  ActionPortLabel=else
  Constant : Constant  Value=0
  F_normal_b : Outport
  wires:
  Constant/1 -> F_normal_b/1

== system Takeoff_Sim/Forces/Normal and Friction/aircraft on ground ==
  F_tot_y : Inport
  Action Port : ActionPort  ActionPortLabel="if(u1 <= 0 & u2 <=  243.661 )"
  Gain : Gain  Gain=-1
  F_normal_b : Outport
  wires:
  F_tot_y/1 -> Gain/1
  Gain/1 -> F_normal_b/1

== system Takeoff_Sim/vel_c to vel_wind/calculate Carrier velocity/If Action Subsystem ==
  Action Port : ActionPort  ActionPortLabel=if(u1 == 1)
  Ground1 : Ground
  Mux : Mux  Inputs=2
  carrier vel : Constant  Value=carrier_vel
  carrier_vel : Outport  PortDimensions=2
  wires:
  carrier vel/1 -> Mux/1
  Ground1/1 -> Mux/2
  Mux/1 -> carrier_vel/1

== system Takeoff_Sim/vel_c to vel_wind/calculate Carrier velocity/If Action Subsystem1 ==
  Action Port : ActionPort  ActionPortLabel=else
  Ground1 : Ground
  Mux : Mux  Inputs=2
  carrier vel : Constant  Value=0
  carrier_vel : Outport  PortDimensions=2
  wires:
  carrier vel/1 -> Mux/1
  Ground1/1 -> Mux/2
  Mux/1 -> carrier_vel/1

== system Takeoff_Sim/Forces/Aerodynamic Forces/Aero Coefficient/Calculate CD ==
  CL : Inport
  Add1 : Sum  Inputs=+++
  CD_0 : Constant  Value=CD_0
  CD_Gear : Constant  Value=CD_LG
  Product1 : Product
  Square : Math  Operator=square
  k_drag : Constant  Value=k_drag
  CD : Outport
  wires:
  Product1/1 -> Add1/2
  CD_0/1 -> Add1/1
  Square/1 -> Product1/2
  CL/1 -> Square/1
  CD_Gear/1 -> Add1/3
  k_drag/1 -> Product1/1
  Add1/1 -> CD/1

== system Takeoff_Sim/Forces/Aerodynamic Forces/Aero Coefficient/Calculate CL ==
  AoA : Inport
  If : If  IfExpression=u1 < 15
  If Action Subsystem : Subsystem  TreatAsAtomicUnit=on
  If Action Subsystem1 : Subsystem  TreatAsAtomicUnit=on
  Merge : Merge
  Radians to Degrees : simulink_extras/Transformations/Radians to Degrees
  CL : Outport
  wires:
  Radians to Degrees/1 -> If/1
  AoA/1 -> If Action Subsystem/1(AoA), Radians to Degrees/1
  If Action Subsystem/1(CL) -> Merge/1
  If Action Subsystem1/1(CL) -> Merge/2
  Merge/1 -> CL/1
  If/1 -> If Action Subsystem/Action
  If/2 -> If Action Subsystem1/Action

== system Takeoff_Sim/Forces/Aerodynamic Forces/Aero Coefficient/Calculate CL/If Action Subsystem ==
  AoA : Inport
  Action Port : ActionPort  ActionPortLabel=if(u1 < 15)
  CL_alpha : Constant  Value=CL_alpha
  Constant : Constant  Value=alpha_L0
  Minus : Sum  Inputs=+-
  Product : Product
  CL : Outport
  wires:
  AoA/1 -> Minus/1
  Constant/1 -> Minus/2
  CL_alpha/1 -> Product/1
  Minus/1 -> Product/2
  Product/1 -> CL/1

== system Takeoff_Sim/Forces/Aerodynamic Forces/Aero Coefficient/Calculate CL/If Action Subsystem1 ==
  Action Port : ActionPort  ActionPortLabel=else
  Constant : Constant  Value=0
  CL : Outport
  wires:
  Constant/1 -> CL/1

== matlab function Takeoff_Sim/predetermined_theta/phase 2: Ramp/MATLAB Function ==
  data: x input; theta output; R input
function theta = fcn(x, R)
    theta = rad2deg(asin((x-200)/R));
end
